simulink model "SimulinkDesign"  (R2024a)
settings: Solver=VariableStepAuto  StartTime=0.0  StopTime=2.5  RelTol=1e-3
libraries: dspfdesign x3, simulink_extras x1, dspsigops x1
settings Model: Creator=sberk019  LastModifiedBy=Tristan Ruel

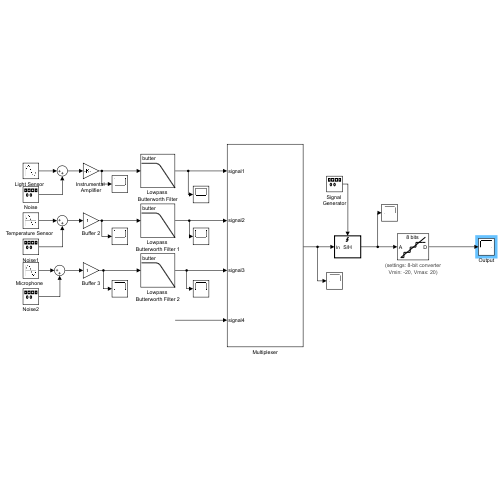
[thumbnail: Simulink's stored preview of the top-level diagram]
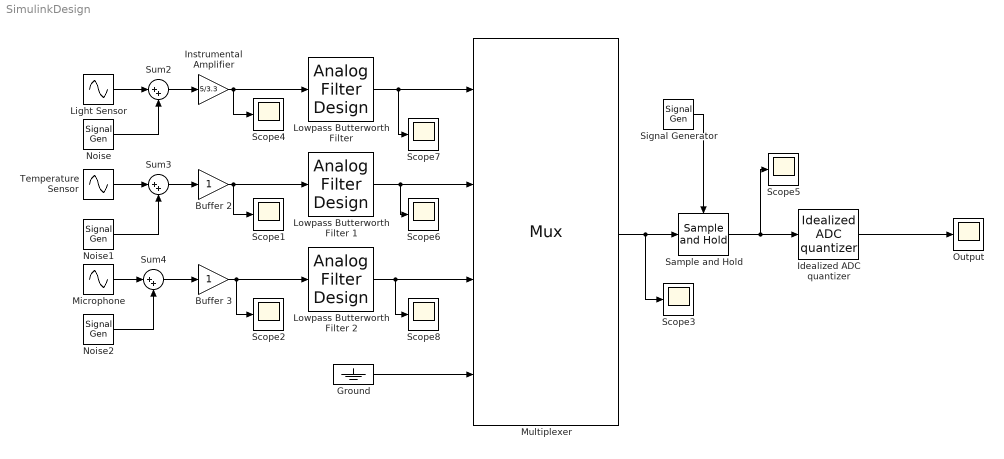
== system SimulinkDesign ==
  Buffer 2 : Gain
  Buffer 3 : Gain
  Ground : Ground
  Idealized ADC quantizer : simulink_extras/Additional Discrete/Idealized ADC quantizer  NumberOfConverterBits=8  Vmin=-20  Vmax=20  OutputDataType=uint8  OutputNegativeValues=off
  Instrumental Amplifier : Gain  Gain=5/3.3
  "Light Sensor  " : Sin  Amplitude=3.3  Frequency=7  SampleTime=0
  Lowpass Butterworth Filter : dspfdesign/Analog Filter Design  method=Butterworth  filttype=Lowpass  N=4  Wlo=25  Whi=80  Rp=2  Rs=40
  Lowpass Butterworth Filter 1 : dspfdesign/Analog Filter Design  method=Butterworth  filttype=Lowpass  N=4  Wlo=25  Whi=80  Rp=2  Rs=40
  Lowpass Butterworth Filter 2 : dspfdesign/Analog Filter Design  method=Butterworth  filttype=Lowpass  N=4  Wlo=25  Whi=80  Rp=2  Rs=40
  "Microphone  " : Sin  Amplitude=5  Frequency=7  SampleTime=0
  Multiplexer : Mux
      settings: DisplayOption=signals
  Noise : SignalGenerator  Frequency=60
  Noise1 : SignalGenerator  Frequency=60
  Noise2 : SignalGenerator  Frequency=60
  Output : Scope
  Sample and Hold : dspsigops/Sample and Hold  trig=Rising edge  initCond=0  latchinput=off
  Scope{1..8} (8 alike) : Scope
  Signal Generator : SignalGenerator  Frequency=100
  Sum2 : Sum  Inputs=|++
  Sum3 : Sum  Inputs=|++
  Sum4 : Sum  Inputs=|++
  "Temperature Sensor  " : Sin  Amplitude=5  Frequency=7  SampleTime=0
  wires:
  Buffer 2/1 -> Scope1/1, Lowpass Butterworth Filter 1/1
  Buffer 3/1 -> Scope2/1, Lowpass Butterworth Filter 2/1
  Lowpass Butterworth Filter 1/1 -> Scope6/1, Multiplexer/2
  Lowpass Butterworth Filter/1 -> Scope7/1, Multiplexer/1
  Multiplexer/1 -> Scope3/1, Sample and Hold/1
  Signal Generator/1 -> Sample and Hold/Trigger
  Sample and Hold/1 -> Scope5/1, Idealized ADC quantizer/1
  Idealized ADC quantizer/1 -> Output/1
  Lowpass Butterworth Filter 2/1 -> Multiplexer/3, Scope8/1
  Ground/1 -> Multiplexer/4
  "Light Sensor  "/1 -> Sum2/1
  Sum2/1 -> Instrumental Amplifier/1
  Sum3/1 -> Buffer 2/1
  Sum4/1 -> Buffer 3/1
  "Microphone  "/1 -> Sum4/1
  "Temperature Sensor  "/1 -> Sum3/1
  Instrumental Amplifier/1 -> Lowpass Butterworth Filter/1, Scope4/1
  Noise/1 -> Sum2/2
  Noise2/1 -> Sum4/2
  Noise1/1 -> Sum3/2
